simulink model "m2_QPSK"  (R2018a)
settings: Solver=VariableStepAuto  StartTime=0.0  StopTime=30  RelTol=1e-3
libraries: commutil2 x5, commseqgen3 x2, commdigbbndpm3 x2, commchan3 x1, commrandsrc3 x1, commsink2 x1
settings Model: Creator=acer  LastModifiedBy=12053

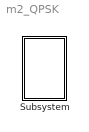
== system m2_QPSK ==
  Subsystem : Subsystem  mask{Parameter1=0}

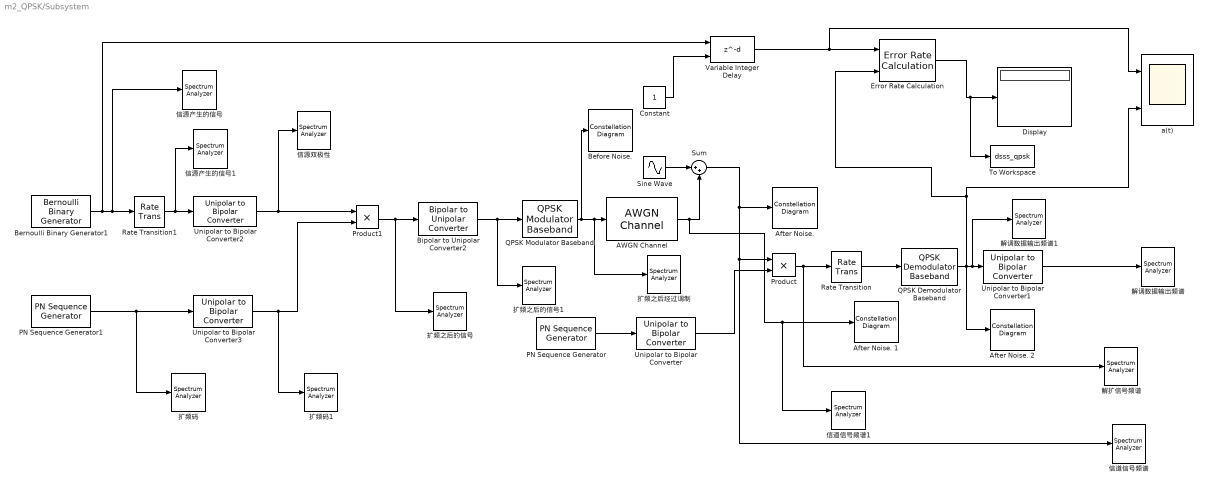
== system m2_QPSK/Subsystem ==
  AWGN Channel : commchan3/AWGN Channel  InputProcessing=Columns as channels (frame based)  seed=0  noiseMode="Signal to noise ratio  (Eb/No)"  EbNodB=0  EsNodB=80  SNRdB=5  bitsPerSym=2  Ps=1e-6  Tsym=0.01  variance=1
  "After Noise. " : ConstellationDiagram
  After Noise. 1 : ConstellationDiagram
  After Noise. 2 : ConstellationDiagram
  Before Noise. : ConstellationDiagram
  Bernoulli Binary Generator1 : commrandsrc3/Bernoulli Binary Generator  ProbabilityOfZero=0.5  SeedSource=Parameter  Seed=63  SampleTime=0.01  SamplesPerFrame=100  OutputDataType=double  SimulateUsing=Interpreted execution
  Bipolar to Unipolar Converter2 : commutil2/Bipolar to Unipolar Converter  M=2  polarity=Positive  dataType=Inherit via internal rule
      settings: SourceProductName=Communications System Toolbox  SourceProductBaseCode=CM
  Constant : Constant
  Display : Display
  Error Rate Calculation : commsink2/Error Rate Calculation  N=0  st_delay=0  cp_mode=Entire frame  subframe=[]  PMode=Port  WsName=ErrorRate  RsMode2=off  stop=off  numErr=100  maxBits=1e6
  PN Sequence Generator : commseqgen3/PN Sequence Generator  poly='z^6 + z + 1'  ini_sta=[0 0 0 0 0 1]  outBitMaskSource=Dialog parameter  shift=0  outVarSiz=off  maxOutSizeMode=Dialog parameter  maxOutSize=[10 1]  Ts=1/2000  sampPerFrame=1  reset=off  bitPackedOutputs=off  outDataType=double  numPackedBits=8  bitPackDataSigned=off  bitPackedOutDType=double
      settings: SourceProductName=Communications System Toolbox
  PN Sequence Generator1 : commseqgen3/PN Sequence Generator  poly='z^6 + z + 1'  ini_sta=[0 0 0 0 0 1]  outBitMaskSource=Dialog parameter  shift=0  outVarSiz=off  maxOutSizeMode=Dialog parameter  maxOutSize=[10 1]  Ts=1/2000  sampPerFrame=1  reset=off  bitPackedOutputs=off  outDataType=double  numPackedBits=8  bitPackDataSigned=off  bitPackedOutDType=double
      settings: SourceProductName=Communications System Toolbox
  Product : Product
  Product1 : Product
  QPSK Demodulator Baseband : commdigbbndpm3/QPSK Demodulator Baseband  OutType=Bit  DecType=Hard decision  VarSource=Dialog  Variance=1  Dec=Gray  Ph=0  outDtype1=Inherit via internal rule  outDtype2=Inherit via internal rule  derotateFactorWordLen=16  derotateFactorDataTypeStr=Inherit: Same word length as input  derotateFactorLastDataTypeStr=Inherit: Same word length as input
  QPSK Modulator Baseband : commdigbbndpm3/QPSK Modulator Baseband  InType=Bit  Enc=Gray  Ph=0  outDtype=double  outWordLen=16  outUDDataType=sfix(16)  outFracLenMode=Best precision  outFracLen=15  outDataTypeStr=double  outLastDataTypeStr=double
  Rate Transition : RateTransition  InitialCondition=1  OutPortSampleTime=1
  Rate Transition1 : RateTransition  Deterministic=off  OutPortSampleTime=1/2000
  Sine Wave : Sin  Frequency=300  SampleTime=1/2000
  Sum : Sum  Inputs=|++
  To Workspace : ToWorkspace  VariableName=dsss_qpsk  SampleTime=-1
      settings: Save2DSignal=2-D array (concatenate along first dimension)
  Unipolar to Bipolar Converter{,1..3} (4 alike) : commutil2/Unipolar to Bipolar Converter  M=2  polarity=Positive  dataType=Inherit via internal rule
      settings: SourceProductName=Communications System Toolbox
  Variable Integer Delay : Delay  DelayLengthSource=Input port
      settings: InputPortMap=u0,p1
  a(t) : Scope  NumInputPorts=2
  信源产生的信号 : SpectrumAnalyzer
  信源产生的信号1 : SpectrumAnalyzer
  信源双极性 : SpectrumAnalyzer
  信道信号频谱 : SpectrumAnalyzer
  信道信号频谱1 : SpectrumAnalyzer
  扩频之后的信号 : SpectrumAnalyzer
  扩频之后的信号1 : SpectrumAnalyzer
  扩频之后经过调制 : SpectrumAnalyzer
  扩频码 : SpectrumAnalyzer
  扩频码1 : SpectrumAnalyzer
  解扩信号频谱 : SpectrumAnalyzer
  解调数据输出频谱 : SpectrumAnalyzer
  解调数据输出频谱1 : SpectrumAnalyzer
  wires:
  Sine Wave/1 -> Sum/1
  PN Sequence Generator/1 -> Unipolar to Bipolar Converter/1
  Unipolar to Bipolar Converter/1 -> Product/2
  Unipolar to Bipolar Converter1/1 -> 解调数据输出频谱/1
  QPSK Modulator Baseband/1 -> Before Noise./1, 扩频之后经过调制/1, AWGN Channel/1
  AWGN Channel/1 -> 信道信号频谱1/1, After Noise. 1/1, Sum/2
  Product/1 -> 解扩信号频谱/1, Rate Transition/1
  Sum/1 -> "After Noise. "/1, 信道信号频谱/1, Product/1
  Bernoulli Binary Generator1/1 -> Variable Integer Delay/1, 信源产生的信号/1, Rate Transition1/1
  Error Rate Calculation/1 -> To Workspace/1, Display/1
  Rate Transition/1 -> QPSK Demodulator Baseband/1
  Variable Integer Delay/1 -> a(t)/1, Error Rate Calculation/1
  QPSK Demodulator Baseband/1 -> After Noise. 2/1, Error Rate Calculation/2, a(t)/2, 解调数据输出频谱1/1, Unipolar to Bipolar Converter1/1
  Constant/1 -> Variable Integer Delay/2
  Unipolar to Bipolar Converter2/1 -> 信源双极性/1, Product1/1
  Rate Transition1/1 -> 信源产生的信号1/1, Unipolar to Bipolar Converter2/1
  PN Sequence Generator1/1 -> 扩频码/1, Unipolar to Bipolar Converter3/1
  Unipolar to Bipolar Converter3/1 -> 扩频码1/1, Product1/2
  Product1/1 -> 扩频之后的信号/1, Bipolar to Unipolar Converter2/1
  Bipolar to Unipolar Converter2/1 -> 扩频之后的信号1/1, QPSK Modulator Baseband/1
